simulink model "PROTOTYPE_SIM"  (R2024b)
settings: Solver=ode15s  StartTime=0.0  StopTime=0.1  FixedStep=1e-8  MaxStep=1e-7  RelTol=1e-3
InitFcn:
  | param = struct();
  | 
  | % Pressure Rails
  | param.P_H = 20e6;
  | param.P_M = 10e6;
  | param.P_L = 101325;
  | 
  | % Linear Actuator Chamber
  | param.V1_0 = 250e-6;
  | param.Acap = pi*(0.5*2.54)^2*1e-4;
  | 
  | % Intermediary volumes
  | param.V3_0 = 10e-6;
  | param.V4_0 = 10e-6;
  | 
  | % Fluid
  | param.beta = 1.8e9;
  | param.air = 5/100;
  | param.rho = 870;
  | 
  | % Valve
  | param.max_Avt = 0.5*0.25*pi*(20e-3)^2;
  | param.Cd = 0.6;
  | 
  | % Valve Dynamics
  | param.wn = 50*2*pi;
  | param.zeta = 1;
  | 
  | % Hydraulic Pump/Motor
  | param.J_hyd = 3000e-7;
  | param.D = 0.8e-6;    % In cc/rev
  | param.pump_mech_eff = 100*(1/100);
  | param.pump_vol_eff = 100*(1/100);
  | 
  | % Electric Motor/Generator
  | param.J_elec = 3060e-7;
  | param.Kt = 109e-3;
  | param.Kv = (88*pi)/30; % In rads^-1/Volt
  | param.elec_eff = 100*(1/100);
  | param.max_mech_power = 90;
settings Model: Creator=user  LastModifiedBy=user

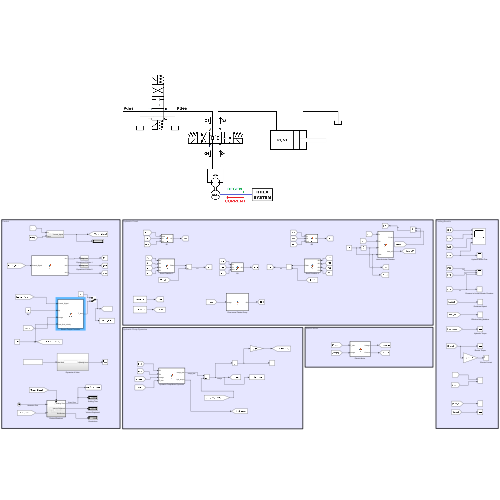
[thumbnail: Simulink's stored preview of the top-level diagram]
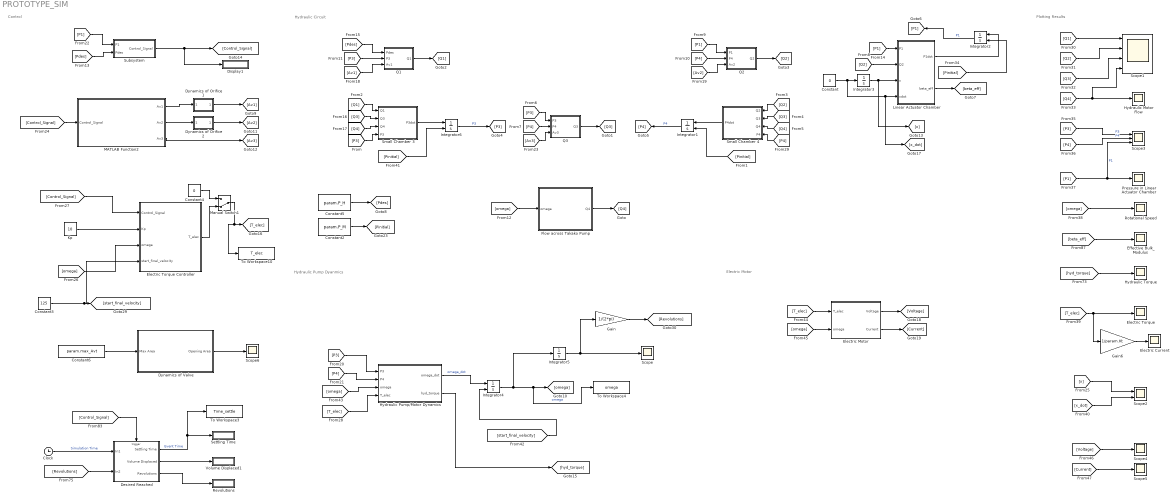
== system PROTOTYPE_SIM ==
  note: Electric Motor
  note: Plotting Results
  note: Hydraulic Pump Dyanmics
  note: Hydraulic Circuit
  note: Control
  Clock : Clock
  Constant : Constant  Value=0
  Constant2 : Constant  Value=param.P_M
  Constant3 : Constant  Value=125
  Constant4 : Constant  Value=0
  Constant5 : Constant  Value=param.P_H
  Constant6 : Constant  Value=param.max_Avt
  Desired Reached : Subsystem  TreatAsAtomicUnit=on
  Display1 : Display
  Dynamics of Orifice 1 : Subsystem
  Dynamics of Orifice 2 : Subsystem
  Dynamics of Valve : Subsystem
  Effective Bulk_Modulus : Scope
  Electric Current : Scope
  Electric Motor : MATLAB Function  TreatAsAtomicUnit=on
  Electric Torque : Scope
  Electric Torque Controller : MATLAB Function  TreatAsAtomicUnit=on
  Flow across Takako Pump : MATLAB Function  TreatAsAtomicUnit=on
  Gain : Gain  Gain=1/(2*pi)
  Gain6 : Gain  Gain=1/param.Kt
  Hydraulic Motor Flow : Scope
  Hydraulic Pump/Motor Dynamics : MATLAB Function  TreatAsAtomicUnit=on
  Hydraulic Torque : Scope
  Integrator1 : Integrator  InitialConditionSource=external  InitialCondition=param.P_M
  Integrator2 : Integrator  InitialConditionSource=external
  Integrator3 : Integrator
  Integrator4 : Integrator  InitialConditionSource=external
  Integrator5 : Integrator
  Integrator6 : Integrator  InitialConditionSource=external  InitialCondition=param.P_M
  Kp : Constant  Value=10
  Linear Actuator Chamber : MATLAB Function  TreatAsAtomicUnit=on
  MATLAB Function2 : MATLAB Function  TreatAsAtomicUnit=on
  Manual Switch1 : ManualSwitch  CurrentSetting=0
  Pressure in Linear Actuator Chamber : Scope
  Q1 : MATLAB Function  TreatAsAtomicUnit=on
  Q2 : MATLAB Function  TreatAsAtomicUnit=on
  Q3 : MATLAB Function  TreatAsAtomicUnit=on
  Revolutions : Display
  Rotational Speed : Scope
  Scope{,4..6} (4 alike) : Scope
  Scope1 : Scope  NumInputPorts=4
  Scope2 : Scope  NumInputPorts=2
  Scope3 : Scope  NumInputPorts=3
  Settling Time : Display
  Small Chamber 3 : MATLAB Function  TreatAsAtomicUnit=on
  Small Chamber 4 : MATLAB Function  TreatAsAtomicUnit=on
  Subsystem : Subsystem
  To Workspace10 : ToWorkspace  VariableName=T_elec  SaveFormat=Timeseries  SampleTime=-1
  To Workspace3 : ToWorkspace  VariableName=Time_settle  SaveFormat=Timeseries  SampleTime=-1
  To Workspace4 : ToWorkspace  VariableName=omega  SaveFormat=Timeseries  SampleTime=-1
  Volume Displaced1 : Display
  wires:
  Q1/1(Q1) -> [Q1]
  Q3/1(Q3) -> [Q3]
  Flow across Takako Pump/1(Q4) -> [Q4]
  Q2/1(Q2) -> [Q2]
  [P3] -> Q3/1(P3)
  [P4] -> Q3/2(P4)
  Linear Actuator Chamber/1(P1dot) -> Integrator2/1
  [Q2] -> Linear Actuator Chamber/2(Q2)
  Integrator3/1 -> [x], Linear Actuator Chamber/3(x)
  Constant/1 -> [x_dot], Linear Actuator Chamber/4(xdot), Integrator3/1
  Integrator2/1 -> [P1]  "P1"
  [P1] -> Q2/1(P1)
  [P4] -> Q2/2(P4)
  [Pdes] -> Q1/1(Pdes)
  [P3] -> Q1/2(P3)
  [T_elec] -> Hydraulic Pump/Motor Dynamics/4(T_elec)
  Hydraulic Pump/Motor Dynamics/1(omega_dot) -> Integrator4/1  "omega_dot"
  Integrator4/1 -> Integrator5/1, To Workspace4/1, [omega]  "omega"
  Hydraulic Pump/Motor Dynamics/2(hyd_torque) -> [hyd_torque]
  Integrator5/1 -> Scope/1, Gain/1
  Gain/1 -> [Revolutions]
  [start_final_velocity] -> Integrator4/2
  [P4] -> Hydraulic Pump/Motor Dynamics/2(P4)
  [P3] -> Hydraulic Pump/Motor Dynamics/1(P3)
  [omega] -> Flow across Takako Pump/1(omega)
  [Q2] -> Scope1/2
  [P1] -> Scope3/3, Pressure in Linear Actuator Chamber/1  "P1"
  [Q3] -> Scope1/3
  [Q4] -> Hydraulic Motor Flow/1, Scope1/4
  Gain6/1 -> Electric Current/1
  [T_elec] -> Electric Torque/1, Gain6/1
  [hyd_torque] -> Hydraulic Torque/1
  [Q1] -> Scope1/1
  [omega] -> Rotational Speed/1
  [beta_eff] -> Effective Bulk_Modulus/1
  [P3] -> Scope3/1  "P3"
  [P4] -> Scope3/2  "P4"
  [Revolutions] -> Desired Reached/2(In2)
  [P1] -> Subsystem/1(P1)
  Desired Reached/3(Revolutions) -> Revolutions/1
  [Pdes] -> Subsystem/2(Pdes)
  Electric Torque Controller/1(T_elec) -> Manual Switch1/2
  Desired Reached/2(Volume Displaced) -> Volume Displaced1/1
  Manual Switch1/1 -> To Workspace10/1, [T_elec]
  [Control_Signal] -> MATLAB Function2/1(Control_Signal)
  Constant4/1 -> Manual Switch1/1
  Subsystem/1(Control_Signal) -> [Control_Signal], Display1/1
  Constant6/1 -> Dynamics of Valve/1(Max Area)
  Kp/1 -> Electric Torque Controller/2(Kp)
  Desired Reached/1(Settling Time) -> Settling Time/1, To Workspace3/1  "Event Time"
  Dynamics of Valve/1(Opening Area) -> Scope6/1
  Constant3/1 -> Electric Torque Controller/4(start_final_velocity), [start_final_velocity]
  Clock/1 -> Desired Reached/1(In1)  "Simulation Time"
  [Control_Signal] -> Electric Torque Controller/1(Control_Signal)
  [Control_Signal] -> Desired Reached/Trigger
  [omega] -> Electric Torque Controller/3(omega)
  [P1] -> Linear Actuator Chamber/1(P1)
  Linear Actuator Chamber/2(beta_eff) -> [beta_eff]
  Constant5/1 -> [Pdes]
  Constant2/1 -> [Pinitial]
  [Av1] -> Q1/3(Av1)
  [Av2] -> Q2/3(Av2)
  [Av3] -> Q3/3(Av3)
  Integrator6/1 -> [P3]  "P3"
  Small Chamber 3/1(P3dot) -> Integrator6/1
  [Pinitial] -> Integrator6/2
  Small Chamber 4/1(P4dot) -> Integrator1/1
  [Pinitial] -> Integrator1/2
  Integrator1/1 -> [P4]  "P4"
  [P3] -> Small Chamber 3/4(P3)
  [Q1] -> Small Chamber 3/1(Q1)
  [Q2] -> Small Chamber 4/1(Q2)
  [Q3] -> Small Chamber 4/2(Q3)
  [Q4] -> Small Chamber 4/3(Q4)
  [Q3] -> Small Chamber 3/2(Q3)
  [Q4] -> Small Chamber 3/3(Q4)
  [P4] -> Small Chamber 4/4(P4)
  [Pinitial] -> Integrator2/2
  Dynamics of Orifice 1/1(Opening Area) -> [Av1]
  Dynamics of Orifice 2/1(Opening Area) -> [Av2]
  MATLAB Function2/3(Av3) -> [Av3]
  MATLAB Function2/1(Av1) -> Dynamics of Orifice 1/1(Max Area)
  MATLAB Function2/2(Av2) -> Dynamics of Orifice 2/1(Max Area)
  [x] -> Scope2/1
  [x_dot] -> Scope2/2
  [omega] -> Hydraulic Pump/Motor Dynamics/3(omega)
  [T_elec] -> Electric Motor/1(T_elec)
  [omega] -> Electric Motor/2(omega)
  Electric Motor/1(Voltage) -> [Voltage]
  Electric Motor/2(Current) -> [Current]
  [Current] -> Scope5/1
  [Voltage] -> Scope4/1

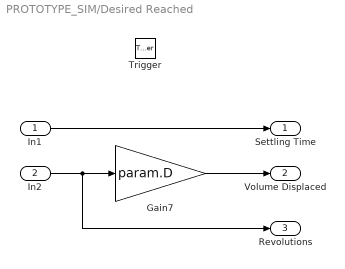
== system PROTOTYPE_SIM/Desired Reached ==
  In1 : Inport
  In2 : Inport  Port=2
  Trigger : TriggerPort  VariantControl=(inherit)
  Gain7 : Gain  Gain=param.D
  Settling Time : Outport
  Volume Displaced : Outport  Port=2
  Revolutions : Outport  Port=3
  wires:
  In1/1 -> Settling Time/1
  Gain7/1 -> Volume Displaced/1
  In2/1 -> Revolutions/1, Gain7/1

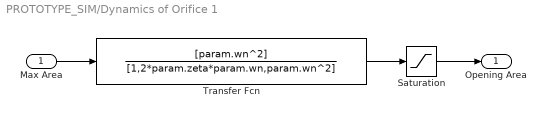
== system PROTOTYPE_SIM/Dynamics of Orifice 1 ==
  Max Area : Inport
  Saturation : Saturate  UpperLimit=param.max_Avt  LowerLimit=0
  Transfer Fcn : TransferFcn  Numerator=[param.wn^2]  Denominator=[1,2*param.zeta*param.wn,param.wn^2]
  Opening Area : Outport
  wires:
  Max Area/1 -> Transfer Fcn/1
  Saturation/1 -> Opening Area/1
  Transfer Fcn/1 -> Saturation/1

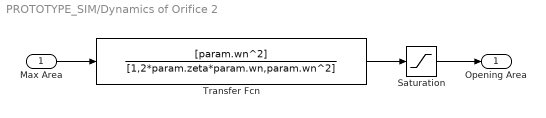
== system PROTOTYPE_SIM/Dynamics of Orifice 2 ==
  Max Area : Inport
  Saturation : Saturate  UpperLimit=param.max_Avt  LowerLimit=0
  Transfer Fcn : TransferFcn  Numerator=[param.wn^2]  Denominator=[1,2*param.zeta*param.wn,param.wn^2]
  Opening Area : Outport
  wires:
  Transfer Fcn/1 -> Saturation/1
  Saturation/1 -> Opening Area/1
  Max Area/1 -> Transfer Fcn/1

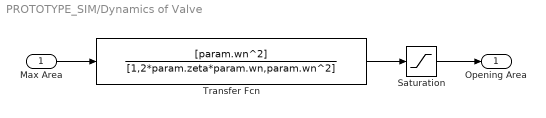
== system PROTOTYPE_SIM/Dynamics of Valve ==
  Max Area : Inport
  Saturation : Saturate  UpperLimit=param.max_Avt  LowerLimit=0
  Transfer Fcn : TransferFcn  Numerator=[param.wn^2]  Denominator=[1,2*param.zeta*param.wn,param.wn^2]
  Opening Area : Outport
  wires:
  Transfer Fcn/1 -> Saturation/1
  Saturation/1 -> Opening Area/1
  Max Area/1 -> Transfer Fcn/1

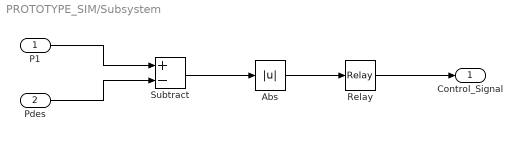
== system PROTOTYPE_SIM/Subsystem ==
  P1 : Inport
  Pdes : Inport  Port=2
  Abs : Abs  SaturateOnIntegerOverflow=off
  Relay : Relay  OnSwitchValue=1e6  OffSwitchValue=1e4  OnOutputValue=0  OffOutputValue=1
  Subtract : Sum  Inputs=+-
  Control_Signal : Outport
  wires:
  P1/1 -> Subtract/1
  Pdes/1 -> Subtract/2
  Subtract/1 -> Abs/1
  Abs/1 -> Relay/1
  Relay/1 -> Control_Signal/1

== matlab function PROTOTYPE_SIM/Hydraulic Pump//Motor Dynamics ==
  data: P3 input; omega_dot output; P4 input; omega input; T_elec input; param parameter; hyd_torque output
function [omega_dot, hyd_torque] = fcn(P3,P4,omega,T_elec,param)

% 1st term for motoring case, 2nd term for pumping case
dP = P3-P4;

hyd_torque = (omega*dP > 0)*(param.D/(2*pi))*(dP)*param.pump_mech_eff +...
    (omega*dP < 0)*(param.D/(2*pi))*(dP)/param.pump_mech_eff;

% hyd_torque = (param.D/(2*pi))*(P3-P4);
omega_dot = (1/(param.J_elec+param.J_hyd))*(hyd_torque-T_elec);

== matlab function PROTOTYPE_SIM/Electric Torque Controller ==
  data: Control_Signal input; Kp input; omega input; T_elec output; start_final_velocity input
function T_elec  = fcn(Control_Signal, Kp, omega, start_final_velocity)


if Control_Signal == 1 
% Phase 2

    if omega < start_final_velocity
        omega_error = -start_final_velocity + omega;
        
        T_elec = Kp*omega_error;
        
    else
        T_elec = 1;
    end

else
% Phase 1

    if omega >= 150
        omega_error = omega - 150;


        T_elec = Kp*omega_error;
       
    else
        T_elec = -1;
    end

end

== matlab function PROTOTYPE_SIM/Small Chamber 4 ==
  data: Q2 input; Q3 input; P4dot output; Q4 input; P4 input; param parameter
function P4dot = fcn(Q2, Q3, Q4, P4, param)

gamma = 1.4; % Adiabatic process
Pt = param.P_L;

Pg = P4-Pt;   % Gauge pressure
r = P4/Pt;    % Pressure ratio
r = abs(r);
e = exp(Pg/param.beta);
rv = (1/e + param.air*r^(-1/gamma))/(1+param.air);      %Volume ratio

% Note: beta_mix as calculated by Hans Barkei
beta_eff = rv*(1+param.air)/(1/(e*param.beta)+param.air/(gamma*Pt*r^(1/gamma+1)));

% beta_eff = param.beta;

P4dot = (beta_eff/(param.V4_0))*(Q3+Q4-Q2);

== matlab function PROTOTYPE_SIM/Q1 ==
  data: Pdes input; Q1 output; P3 input; Av1 input; param parameter
function Q1 = fcn(Pdes, P3, Av1, param)

P_diff = Pdes - P3;
Q1 = param.Cd*Av1*sqrt(2/param.rho)*sqrt(abs(P_diff))*sign(P_diff);

== matlab function PROTOTYPE_SIM/Q3 ==
  data: P3 input; P4 input; Av3 input; Q3 output; param parameter
function Q3 = fcn(P3, P4, Av3, param)

P_diff = P3 - P4;
Q3 = param.Cd*Av3*sqrt(2/param.rho)*sqrt(abs(P_diff))*sign(P_diff);

== matlab function PROTOTYPE_SIM/Flow across Takako Pump ==
  data: omega input; Q4 output; param parameter
function Q4 = fcn(omega, param)

Q4 = (param.pump_vol_eff)*(param.D/(2*pi))*omega;

== matlab function PROTOTYPE_SIM/Small Chamber 3 ==
  data: Q1 input; Q3 input; P3dot output; Q4 input; P3 input; param parameter
function P3dot = fcn(Q1, Q3, Q4, P3, param)

gamma = 1.4; % Adiabatic process
Pt = param.P_L;

Pg = P3-Pt;   % Gauge pressure
r = P3/Pt;    % Pressure ratio
r = abs(r);
e = exp(Pg/param.beta);
rv = (1/e+param.air*r^(-1/gamma))/(1+param.air);      %Volume ratio

% Note: beta_mix as calculated by Hans Barkei
beta_eff = rv*(1+param.air)/(1/(e*param.beta)+param.air/(gamma*Pt*r^(1/gamma+1)));

% beta_eff = param.beta;

P3dot = (beta_eff/(param.V3_0))*(Q1-Q3-Q4);

== matlab function PROTOTYPE_SIM/Q2 ==
  data: P1 input; Q2 output; P4 input; Av2 input; param parameter
function Q2 = fcn(P1, P4, Av2, param)

P_diff = P4-P1;
Q2 = param.Cd*Av2*sqrt(2/param.rho)*sqrt(abs(P_diff))*sign(P_diff);

== matlab function PROTOTYPE_SIM/MATLAB Function2 ==
  data: Control_Signal input; Av1 output; param parameter; Av2 output; Av3 output
function [Av1, Av2, Av3] = fcn(Control_Signal, param)

if Control_Signal==1
    
    % Phase 2
    Av1 = param.max_Avt;
    Av2 = param.max_Avt;
    Av3 = param.max_Avt;

else

    % Phase 1
    Av1 = param.max_Avt;
    Av2 = param.max_Avt;
    Av3 = 0;

end

== matlab function PROTOTYPE_SIM/Electric Motor ==
  data: T_elec input; Voltage output; omega input; param parameter; Current output
function [Voltage, Current] = fcn(T_elec, omega, param)

Mech_Power = T_elec*omega;

if (Mech_Power < param.max_mech_power)
    
    Current = (T_elec/param.Kt);
    Voltage = (omega/param.Kv);

else

    Current = (T_elec/param.Kt);
    Voltage = (param.max_mech_power/Current);
    
end

== matlab function PROTOTYPE_SIM/Linear Actuator Chamber ==
  data: P1 input; Q2 input; P1dot output; x input; xdot input; param parameter; beta_eff output
function [P1dot, beta_eff] = fcn(P1,Q2,x, xdot, param)

gamma = 1.4; % Adiabatic process
Pt = param.P_L;

Pg = P1-Pt;   % Gauge pressure
r = P1/Pt;    % Pressure ratio
r = abs(r);
e = exp(Pg/param.beta);
rv = (1/e+param.air*r^(-1/gamma))/(1+param.air);      %Volume ratio

% Note: beta_mix as calculated by Hans Barkei
beta_eff = rv*(1+param.air)/(1/(e*param.beta)+param.air/(gamma*Pt*r^(1/gamma+1)));

% beta_eff = param.beta;

P1dot = (beta_eff/(param.V1_0+param.Acap*x))*(Q2-param.Acap*xdot);
